simulink model "LQGn"  (R2024a)
settings: Solver=VariableStepAuto  StartTime=0.0  StopTime=10.0  RelTol=1e-6
values from neighbouring files (symbols this model uses):
  A = [0, 1, 0, 0 ... (first row only)    [get_matrices.m]    (also in main.m)
  B = [0; 4 / (4 * M + m); 0; 3 / (l * (4 * M + m))]    [get_matrices.m]    (also in main.m = [0; 0; 1 / M; -1 / (l * M)])
  C = [1, 0, 0, 0; 0, 0, 1, 0]    [get_matrices.m]    (also in main.m)
  K = -R \ B' * P    [TAU.m]    (also in chapter3.m = TAU.FindControllerSylvester(A, B, GammaK); chapter4.m = pairs{i}{1}; chapter6.m = TAU.FindControllerLMI(A, B, 2); main.m = FindControllerSylvester(A, B, Gamma))
  l = l / 2    [get_initials.m]    (also in main.m)
  L = -P * C' / R    [TAU.m]    (also in chapter4.m = pairs{i}{2}; chapter6.m = TAU.FindObserverKalman(A, C, Q, R))
  M = randi([100000 1000000]) / 1000 / sqrt(2)    [get_initials.m]    (also in main.m)
  m = randi([1000 10000]) / 1000 * sqrt(3)    [get_initials.m]    (also in main.m)
  theta0 = 0.1    [chapter2.m]    (also in chapter3.m; chapter4.m = 0.2; chapter5.m = 0.2; chapter6.m = 0.2)
  vare = 0.06    [chapter6.m]
  varf = 0.1    [chapter6.m]
settings Model: Creator=alexivanov  LastModifiedBy=alexivanov

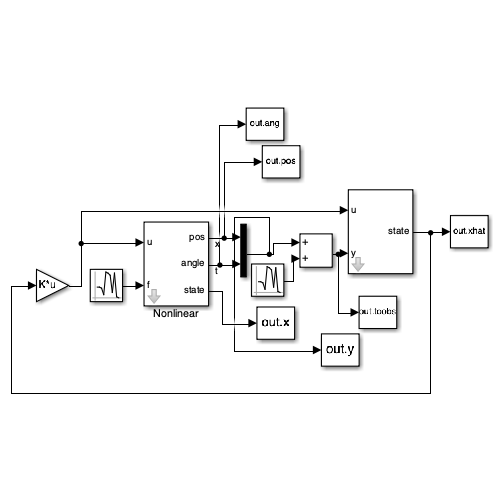
[thumbnail: Simulink's stored preview of the top-level diagram]
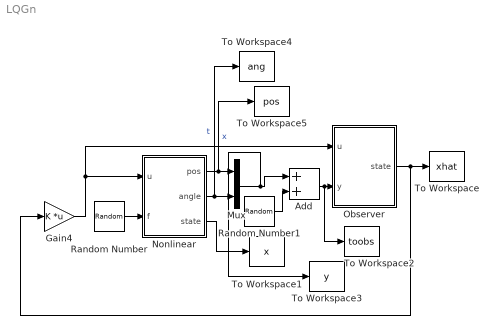
== system LQGn ==
  Add : Sum
  Gain4 : Gain  Gain=K  Multiplication=Matrix(K*u)
  Mux : Mux  Inputs=2
  Nonlinear : Subsystem  mask{Mcart=M, m=m, l=l, g=9.81, theta0=theta0}
      mask prompts: Mcart "Mass of cart (kg)"; m "Mass of pend (kg)"; l "Length of pend (m)"; theta0 "Initial angle (rad)"
  Observer : Subsystem  mask{Mcart=M, m=m, l=l, g=9.81, theta0=theta0}
      mask prompts: Mcart "Mass of cart (kg)"; m "Mass of pend (kg)"; l "Length of pend (m)"; theta0 "Initial angle (rad)"
  Random Number : RandomNumber  Variance=varf  SampleTime=0.001
  Random Number1 : RandomNumber  Variance=vare  SampleTime=0.001
  To Workspace : ToWorkspace  VariableName=xhat  SampleTime=-1
  To Workspace1 : ToWorkspace  VariableName=x  SampleTime=-1
  To Workspace2 : ToWorkspace  VariableName=toobs  SampleTime=-1
  To Workspace3 : ToWorkspace  VariableName=y  SampleTime=-1
  To Workspace4 : ToWorkspace  VariableName=ang  SampleTime=-1
  To Workspace5 : ToWorkspace  VariableName=pos  SampleTime=-1
  wires:
  Gain4/1 -> Nonlinear/1(u), Observer/1(u)
  Observer/1(state) -> Gain4/1, To Workspace/1
  Add/1 -> To Workspace2/1, Observer/2(y)
  Random Number/1 -> Nonlinear/2(f)
  Random Number1/1 -> Add/2
  Nonlinear/1(pos) -> To Workspace5/1, Mux/1  "x"
  Mux/1 -> To Workspace3/1, Add/1
  Nonlinear/3(state) -> To Workspace1/1
  Nonlinear/2(angle) -> To Workspace4/1, Mux/2  "t"

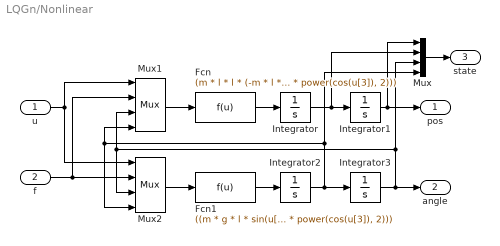
== system LQGn/Nonlinear ==
  u : Inport
  f : Inport  Port=2
  Fcn : Fcn  Expr=(m * l * l * (-m * l * power(u[4], 2) * sin(u[3]) + u[1]) + m * l * cos(u[3]) * (m * g * l * sin(u[3]) + u[2])) / (m * l * l * (Mcart + m - m * power(cos(u[3]), 2)))
  Fcn1 : Fcn  Expr=((m * g * l * sin(u[3]) + u[2]) * (Mcart + m) + m * l * cos(u[3]) * (-m * l * power(u[4], 2) * sin(u[3]) + u[1])) / (m * l * l * (Mcart + m - m * power(cos(u[3]), 2)))
  Integrator : Integrator
  Integrator1 : Integrator
  Integrator2 : Integrator
  Integrator3 : Integrator  InitialCondition=theta0
  Mux : Mux
  Mux1 : Mux
  Mux2 : Mux
  pos : Outport
  angle : Outport  Port=2
  state : Outport  Port=3
  wires:
  Integrator1/1 -> Mux/1, pos/1
  Integrator/1 -> Mux/2, Integrator1/1
  Integrator2/1 -> Mux/4, Mux1/4, Mux2/4, Integrator3/1
  Integrator3/1 -> Mux/3, Mux2/3, Mux1/3, angle/1
  Fcn/1 -> Integrator/1
  u/1 -> Mux2/1, Mux1/1
  f/1 -> Mux2/2, Mux1/2
  Fcn1/1 -> Integrator2/1
  Mux2/1 -> Fcn1/1
  Mux1/1 -> Fcn/1
  Mux/1 -> state/1

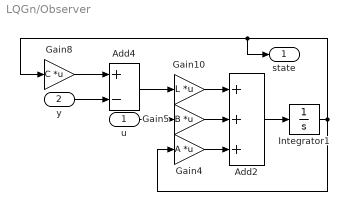
== system LQGn/Observer ==
  u : Inport
  y : Inport  Port=2
  Add2 : Sum  Inputs=+++
  Add4 : Sum  Inputs=+-
  Gain10 : Gain  Gain=L  Multiplication=Matrix(K*u)
  Gain4 : Gain  Gain=A  Multiplication=Matrix(K*u)
  Gain5 : Gain  Gain=B  Multiplication=Matrix(K*u)
  Gain8 : Gain  Gain=C  Multiplication=Matrix(K*u)
  Integrator1 : Integrator
  state : Outport
  wires:
  u/1 -> Gain5/1
  Gain4/1 -> Add2/3
  Gain8/1 -> Add4/1
  Integrator1/1 -> Gain4/1, state/1, Gain8/1
  Add2/1 -> Integrator1/1
  Gain10/1 -> Add2/1
  Add4/1 -> Gain10/1
  y/1 -> Add4/2
  Gain5/1 -> Add2/2
